simulink model "zad3"  (R2022b)
settings: Solver=FixedStepAuto  StartTime=0.0  StopTime=10.0  FixedStep=0.00001  RelTol=1e-3
settings Model: Creator=vandm  LastModifiedBy=vandm

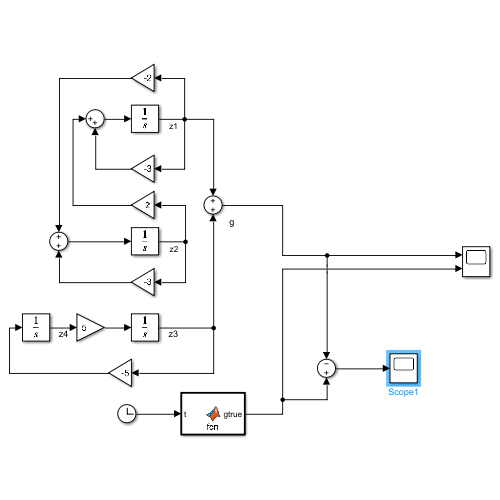
[thumbnail: Simulink's stored preview of the top-level diagram]
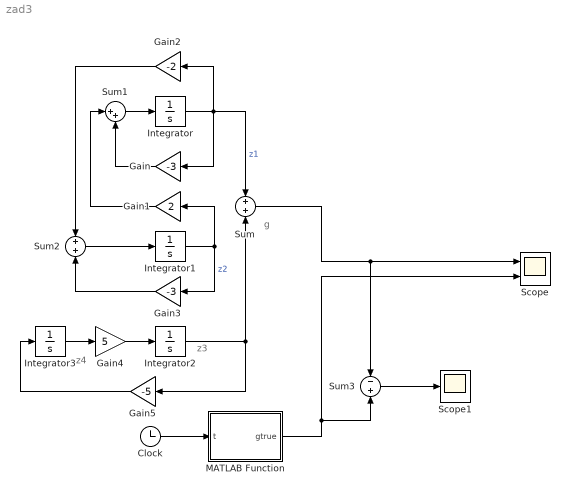
== system zad3 ==
  note: z3
  note: z4
  note: g
  Clock : Clock
  Gain : Gain  Gain=-3
  Gain1 : Gain  Gain=2
  Gain2 : Gain  Gain=-2
  Gain3 : Gain  Gain=-3
  Gain4 : Gain  Gain=5
  Gain5 : Gain  Gain=-5
  Integrator : Integrator
  Integrator1 : Integrator  InitialCondition=3
  Integrator2 : Integrator
  Integrator3 : Integrator  InitialCondition=1.5
  MATLAB Function : MATLAB Function  TreatAsAtomicUnit=on
  Scope : Scope  NumInputPorts=2
  Scope1 : Scope
  Sum : Sum  Inputs=+|+
  Sum1 : Sum  Inputs=|++
  Sum2 : Sum  Inputs=+|+
  Sum3 : Sum  Inputs=-|+
  wires:
  Integrator/1 -> Gain2/1, Gain/1, Sum/1  "z1"
  Gain/1 -> Sum1/2
  Sum1/1 -> Integrator/1
  Integrator1/1 -> Gain3/1, Gain1/1  "z2"
  Gain1/1 -> Sum1/1
  Sum2/1 -> Integrator1/1
  Gain2/1 -> Sum2/1
  Gain3/1 -> Sum2/2
  Integrator2/1 -> Gain5/1, Sum/2
  Integrator3/1 -> Gain4/1
  Gain4/1 -> Integrator2/1
  Gain5/1 -> Integrator3/1
  Sum/1 -> Sum3/1, Scope/1
  Clock/1 -> MATLAB Function/1(t)
  MATLAB Function/1(gtrue) -> Sum3/2, Scope/2
  Sum3/1 -> Scope1/1

== matlab function zad3/MATLAB Function ==
  data: t input; gtrue output
function gtrue = fcn(t)

gtrue = 3 * exp(-3 * t) * sin(2 * t) + 1.5 * sin(5 * t);
